simulink model "ProyectoGlobal_AyCD_Cantu_LagoTejo_OPCUA"  (R2021a)
settings: Solver=ode23  StartTime=0.0  StopTime=inf  MinStep=1e-4
undefined symbols (not defined in the file): a_hMax, a_tMax, b_cx, b_cy, b_eq_h, b_eq_t, b_hb, b_hEb, b_t, b_tb, b_tw, b_wu, bah, bat, bcx, bcy, CI_h, CI_t, Cond_Ini_h, Cond_Ini_t, g, H_c, i_h, i_t, k_cy, k_tw, k_wu, Kcy, Kd_bal, Kp_bal, ksah, ksat, ksiah, ksiat, lim_xDer, lim_xDer_ult, lim_xIzq, lim_xIzq_ult, lim_yInf, lim_yInf_ult, lim_ySup, lim_ySup_ult, M_cMax, M_cMin, M_eq_h, M_eq_t, M_s, M_t, r_hd, r_td, T_hbMax, T_hEbMax, T_hmMax, T_tbMax, T_tmMax, tau_hm, tau_tm, v_hMax_0, v_tMax, xc ... (+2)
libraries: simulink x13, opclib x3
(part 3 of 3)

== matlab function ProyectoGlobal_AyCD_Cantu_LagoTejo_OPCUA/MATLAB Function2 ==
  data: clock input; ON_OFF input; BTN_EMERGENCIA input; Manual input; Ciclo input; max_masa input; Tension_hw input; lim_v_h input; Balanceo input; manual_auto input; ml_medida input; xc input; yc input; graficar input; x_l input; y_l input; x_td input
function grafico_puerto(clock, ON_OFF, BTN_EMERGENCIA, Manual, Ciclo, max_masa, Tension_hw, lim_v_h, Balanceo, manual_auto, ml_medida, xc, yc, graficar, x_l, y_l, x_td)
if(graficar==1)
    alt_txt = 14;   color_cont = "#90AC50";
    fh = figure(100);
    %fh.WindowState = 'maximized';
    clf(fh);
    %figure(100);
    title('Simulación Visual en Tiempo "Real"'),    grid on
    rectangle('Position',[-30, 46, 80, 4],'FaceColor', '#EEEEEE','EdgeColor','#EEEEEE')
    rectangle('Position',[-30, -20, 30, 20],'FaceColor', 'w')
    line([-30 0],[-0.5 -0.5],'Color','black','LineWidth', 5)                    %%% Muelle
    rectangle('Position',[-0.5, 0, 0.5, 15],'FaceColor','black');               %%% Sill Beam
    rectangle('Position',[0.5, -20, 49.5, 25],'EdgeColor','b','LineWidth', 1.5);%%% Barco
    rectangle('Position',[-30, 45, 80, 2],'FaceColor',[0.8 0.8 1]);             %%% Grúa
    rectangle('Position',[x_l-1.25,y_l,2.5,0.5],'FaceColor','k');               %%% Spreader
    rectangle('Position',[x_td-2.5, 45, 5, 2],'FaceColor','k');              %%% Carro
    line([x_l x_td], [y_l 45],'Color','black','LineWidth',2)                 %%% Cable

    for i=1:length(yc)                  %%% Perfil de Carga
        if (xc(i)<2.5)                  %%% Lado de Muelle
            rectangle('Position',[xc(i)-1.25,0,2.5,yc(i)],'FaceColor', color_cont,'LineWidth', 0.3);
        elseif(xc(i)>2.5 && xc(i)<47.5) %%% Lado de Barco
            rectangle('Position',[xc(i)-1.25,-20,2.5,yc(i)+20],'FaceColor', color_cont,'LineWidth', 0.3);
        end
    end

    txt000 = {'Tiempo: ', clock};       %%% Tiempo de Ejecución "Real"
    text(-10, -3.5, txt000,'FontSize', alt_txt)

    if(ON_OFF)                          %%% Cartel de ON - OFF
        txt00 = {'ON: Encendido'};
        text(-30,48.5,txt00,'FontSize',alt_txt,'Color',"#00AA00")
    else
        txt00 = {'OFF: APAGADO'};
        text(-30,48.5,txt00,'FontSize',alt_txt,'Color',"#FF0000")
    end
    
    txt = {'Masa(kg): ', ml_medida};               %%% Cartel de Masa Total en Spreader
    text(-29.75,-17,txt,'FontSize',alt_txt)

    if (ml_medida > 15000)                       %%% Cartel de Cargado/Sin Carga/SOBRECARGA
        rectangle('Position',[x_l-1.25,y_l-2.5,2.5,2.5],'FaceColor', color_cont,'LineWidth', 0.3); %carga
        if (max_masa)
            txt01 = {'SOBRECARGA'};
            text(-22,-17,txt01,'Color','red','FontSize',alt_txt+2)
        else
            txt01 = {'Cargado'};
            text(-22,-17,txt01,'Color',"#00AA00",'FontSize',alt_txt)
        end
    else
        txt01 = {'Sin Carga'};
        text(-22,-17,txt01,'Color',"#CB7A00",'FontSize',alt_txt)
    end

    if (Manual)                       %%% Cartel de Modo de Control
        txt02 = {'Manual'};
        text(-15, 48.5,txt02,'FontSize', alt_txt)
    else
        if (manual_auto)
            txt02 = {'Automático'};
            text(-15, 48.5,txt02,'FontSize',alt_txt)
        else
            txt02 = {'Manual'};
            text(-15, 48.5,txt02,'FontSize',alt_txt)
        end
    end

    if (Balanceo)                       %%% Cartel de Control de Balanceo
        txt03 = {'Balanceo: ON'};
        text(-4, 48.5, txt03,'FontSize',alt_txt,'Color',"#00AA00")
    else
        txt03 = {'Balanceo: OFF'};
        text(-4, 48.5,txt03,'FontSize', alt_txt,'Color','#FF0000')
    end

    if (Tension_hw)                     %%% Cartel de Spreader Apoyado o Suspendido
        txt04 = {'Suspendido'};
        text(10,48.5,txt04,'FontSize', alt_txt)
    else
        txt04 = {'Apoyado'};
        text(10,48.5,txt04,'FontSize', alt_txt)
    end

    if (Ciclo)                          %%% Cartel de Tipo de Ciclo
        txt05 = {'Ciclo Doble'};
        text(22,48.5,txt05,'FontSize', alt_txt)
    else
        txt05 = {'Ciclo Simple'};
        text(22,48.5,txt05,'FontSize', alt_txt)
    end
    
    if (BTN_EMERGENCIA)                 %%% Cartel de EMERGENCIA (botón)
        txt7 = {'EMERGENCIA'};
        rectangle('Position',[34.5, 47, 15.5, 3],'FaceColor', 'red')
        text(35.5,48.5,txt7,'FontSize', alt_txt+6,'Color',"w")
    else
        txt7 = {'OK'};
        rectangle('Position',[34.5, 47, 15.5, 3],'FaceColor', "#00FF00")
        text(41,48.5,txt7,'FontSize', alt_txt+6,'Color',"k")
    end
  
    txt1 = {'Carro (X): ',x_td};                %%% Posiciones del Carro
    text(-29.75,-3.5,txt1,'FontSize',alt_txt)
    txt1 = {'Carro (Y): ',45};
    text(-20,-3.5,txt1,'FontSize',alt_txt)
    txt1 = {'Spreader (X): ',x_l};              %%% Posiciones del Spreader
    text(-29.75,-10,txt1,'FontSize',alt_txt)
    txt1 = {'Spreader (Y): ',y_l};
    text(-20,-10,txt1,'FontSize',alt_txt)
end
end
